simulink model "Task_7"  (R2015a)
settings: Solver=ode45  StartTime=0.0  StopTime=10.0  RelTol=1e-3
undefined symbols (not defined in the file): x
settings Model: Creator=acer  LastModifiedBy=acer

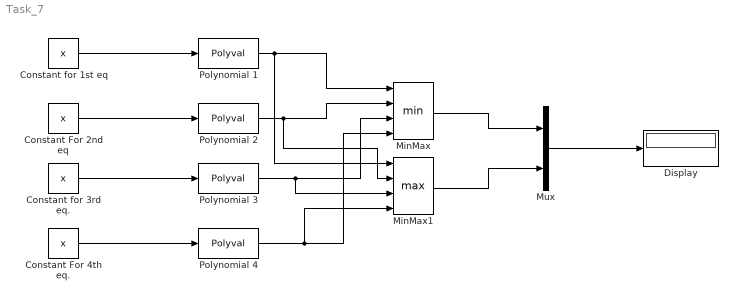
== system Task_7 ==
  Constant For 2nd eq : Constant  Value=x
  Constant For 4th eq. : Constant  Value=x
  Constant for 1st eq : Constant  Value=x
  Constant for 3rd eq. : Constant  Value=x
  Display : Display
  MinMax : MinMax  Inputs=4
  MinMax1 : MinMax  Function=max  Inputs=4
  Mux : Mux  Inputs=2
  Polynomial 1 : Polyval  Coefs=[ 1 0 4 2 7 1 ]
  Polynomial 2 : Polyval  Coefs=[ 4 2 0 0 0]
  Polynomial 3 : Polyval  Coefs=[2 4 6 0 7 1]
  Polynomial 4 : Polyval  Coefs=[ 9 0 2 0 0]
  wires:
  Constant for 1st eq/1 -> Polynomial 1/1
  Constant For 2nd eq/1 -> Polynomial 2/1
  Constant for 3rd eq./1 -> Polynomial 3/1
  Constant For 4th eq./1 -> Polynomial 4/1
  Mux/1 -> Display/1
  Polynomial 1/1 -> MinMax1/1, MinMax/1
  Polynomial 2/1 -> MinMax1/2, MinMax/2
  Polynomial 3/1 -> MinMax1/3, MinMax/3
  Polynomial 4/1 -> MinMax1/4, MinMax/4
  MinMax/1 -> Mux/1
  MinMax1/1 -> Mux/2
